simulink model "OL_HiLData"  (R2015b)
settings: Solver=FixedStepDiscrete  StartTime=0.0  StopTime=stop_time  FixedStep=step_size  RelTol=1e-3
values from neighbouring files (symbols this model uses):
  step_size = 0.1    [loadCalib.m]
  stop_time = 660    [run_test_cases.m]
undefined symbols (not defined in the file or in its folder): canChannel
libraries: canmsglib x62, canlib x29, realtime_pacer_lib x1
(part 3 of 4)

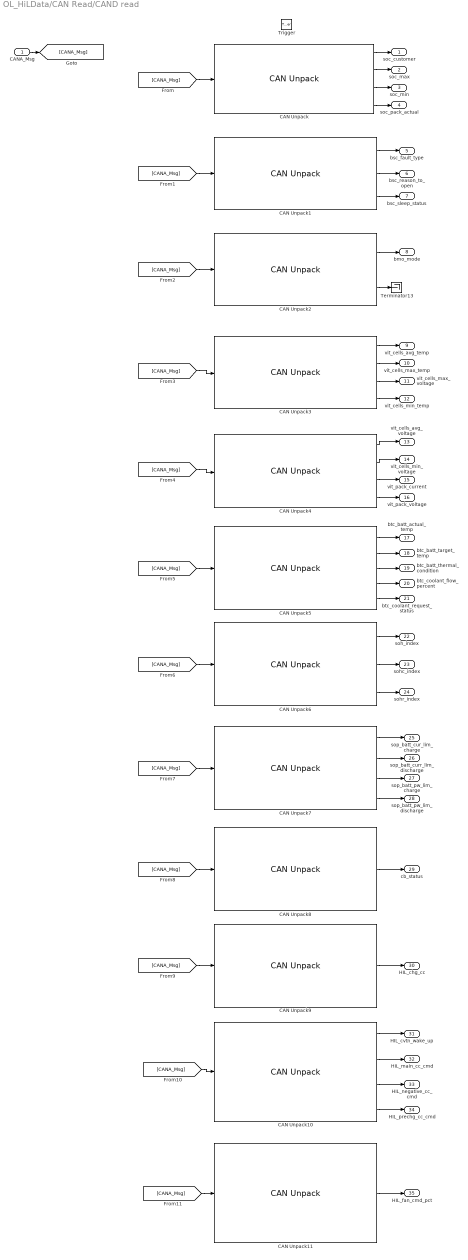
== system OL_HiLData/CAN Read/CAND read ==
  CANA_Msg : Inport
  Trigger : TriggerPort  TriggerType=function-call  PortDimensions=1
  CAN Unpack : canmsglib/CAN Unpack  CANdbFile=D:\Projects\BMS\P006n\08_Work_in_progress\Repo_Sync_folder\OpenLoopDataSendCAN\VEHdb.dbc  MsgList=soc_info  MsgName=soc_info  MsgIDType=Standard (11-bit identifier)  MsgIdentifier=40  MsgLength=8  SignalInfo=soc_customer$8$16$2$2$1$0$1.000000e-02$0$0$100$#soc_max$56$16$2$2$1$0$1.000000e-02$0$0$100$#soc_min$40$16$2$2$1$0$1.000000e-02$0$0$100$#soc_pack_actual$24$16$2$2$1$0$1.000000e-02$0$0$100$#  NSignals=4  IDPort=off  TimestampPort=off  ErrorPort=off  RemotePort=off  LengthPort=off  StatusPort=off  StartBits=str2num('[int32(8);int32(56);int32(40);int32(24)]')  SignalSizes=str2num('[int32(16);int32(16);int32(16);int32(16)]')  ByteOrders=str2num('[int32(2);int32(2);int32(2);int32(2)]')  DataTypes=str2num('[int32(2);int32(2);int32(2);int32(2)]')  MultiplexTypes=str2num('[int32(1);int32(1);int32(1);int32(1)]')  MultiplexValues=str2num('[double(0);double(0);double(0);double(0)]')  Factors=str2num('[double(1.000000e-02);double(1.000000e-02);double(1.000000e-02);double(1.000000e-02)]')  Offsets=str2num('[double(0);double(0);double(0);double(0)]')  Minimums=str2num('[double(0);double(0);double(0);double(0)]')  Maximums=str2num('[double(100);double(100);double(100);double(100)]')
      settings: DataFormat=CANdb specified signals
  CAN Unpack1 : canmsglib/CAN Unpack  CANdbFile=D:\Projects\BMS\P006n\08_Work_in_progress\Repo_Sync_folder\OpenLoopDataSendCAN\VEHdb.dbc  MsgList=bsc_info  MsgName=bsc_info  MsgIDType=Standard (11-bit identifier)  MsgIdentifier=41  MsgLength=8  SignalInfo=bsc_fault_type$8$8$2$2$1$0$1$0$0$20$#bsc_reason_to_open$0$8$2$2$1$0$1$0$0$20$#bsc_sleep_status$23$1$2$2$1$0$1$0$0$1$#  NSignals=3  IDPort=off  TimestampPort=off  ErrorPort=off  RemotePort=off  LengthPort=off  StatusPort=off  StartBits=str2num('[int32(8);int32(0);int32(23)]')  SignalSizes=str2num('[int32(8);int32(8);int32(1)]')  ByteOrders=str2num('[int32(2);int32(2);int32(2)]')  DataTypes=str2num('[int32(2);int32(2);int32(2)]')  MultiplexTypes=str2num('[int32(1);int32(1);int32(1)]')  MultiplexValues=str2num('[double(0);double(0);double(0)]')  Factors=str2num('[double(1);double(1);double(1)]')  Offsets=str2num('[double(0);double(0);double(0)]')  Minimums=str2num('[double(0);double(0);double(0)]')  Maximums=str2num('[double(20);double(20);double(1)]')
      settings: DataFormat=CANdb specified signals
  CAN Unpack10 : canmsglib/CAN Unpack  CANdbFile=D:\Projects\BMS\P006n\08_Work_in_progress\Repo_Sync_folder\OpenLoopDataSendCAN\BMSdb.dbc  MsgList=contactor_cmds  MsgName=contactor_cmds  MsgIDType=Standard (11-bit identifier)  MsgIdentifier=38  MsgLength=8  SignalInfo=cvtn_wake_up$4$1$2$2$1$0$1$0$0$1$#main_contactor_cmd$7$1$2$2$1$0$1$0$0$1$#negative_contactor_cmd$5$1$2$2$1$0$1$0$0$1$#precharge_contactor_cmd$6$1$2$2$1$0$1$0$0$1$#  NSignals=4  IDPort=off  TimestampPort=off  ErrorPort=off  RemotePort=off  LengthPort=off  StatusPort=off  StartBits=str2num('[int32(4);int32(7);int32(5);int32(6)]')  SignalSizes=str2num('[int32(1);int32(1);int32(1);int32(1)]')  ByteOrders=str2num('[int32(2);int32(2);int32(2);int32(2)]')  DataTypes=str2num('[int32(2);int32(2);int32(2);int32(2)]')  MultiplexTypes=str2num('[int32(1);int32(1);int32(1);int32(1)]')  MultiplexValues=str2num('[double(0);double(0);double(0);double(0)]')  Factors=str2num('[double(1);double(1);double(1);double(1)]')  Offsets=str2num('[double(0);double(0);double(0);double(0)]')  Minimums=str2num('[double(0);double(0);double(0);double(0)]')  Maximums=str2num('[double(1);double(1);double(1);double(1)]')
      settings: DataFormat=CANdb specified signals
  CAN Unpack11 : canmsglib/CAN Unpack  CANdbFile=D:\Projects\BMS\P006n\08_Work_in_progress\Repo_Sync_folder\OpenLoopDataSendCAN\BMSdb.dbc  MsgList=fan_cmd  MsgName=fan_cmd  MsgIDType=Standard (11-bit identifier)  MsgIdentifier=39  MsgLength=8  SignalInfo=fan_cmd_pct$14$10$2$2$1$0$1.000000e-01$0$0$100$#  NSignals=1  IDPort=off  TimestampPort=off  ErrorPort=off  RemotePort=off  LengthPort=off  StatusPort=off  StartBits=str2num('[int32(14)]')  SignalSizes=str2num('[int32(10)]')  ByteOrders=str2num('[int32(2)]')  DataTypes=str2num('[int32(2)]')  MultiplexTypes=str2num('[int32(1)]')  MultiplexValues=str2num('[double(0)]')  Factors=str2num('[double(1.000000e-01)]')  Offsets=str2num('[double(0)]')  Minimums=str2num('[double(0)]')  Maximums=str2num('[double(100)]')
      settings: DataFormat=CANdb specified signals
  CAN Unpack2 : canmsglib/CAN Unpack  CANdbFile=D:\Projects\BMS\P006n\08_Work_in_progress\Repo_Sync_folder\OpenLoopDataSendCAN\VEHdb.dbc  MsgList=bmo_info  MsgName=bmo_info  MsgIDType=Standard (11-bit identifier)  MsgIdentifier=48  MsgLength=8  SignalInfo=bmo_mode$0$8$2$2$1$0$1$0$0$10$#soc_rate_high$15$1$2$2$1$0$1$0$0$1$#  NSignals=2  IDPort=off  TimestampPort=off  ErrorPort=off  RemotePort=off  LengthPort=off  StatusPort=off  StartBits=str2num('[int32(0);int32(15)]')  SignalSizes=str2num('[int32(8);int32(1)]')  ByteOrders=str2num('[int32(2);int32(2)]')  DataTypes=str2num('[int32(2);int32(2)]')  MultiplexTypes=str2num('[int32(1);int32(1)]')  MultiplexValues=str2num('[double(0);double(0)]')  Factors=str2num('[double(1);double(1)]')  Offsets=str2num('[double(0);double(0)]')  Minimums=str2num('[double(0);double(0)]')  Maximums=str2num('[double(10);double(1)]')
      settings: DataFormat=CANdb specified signals
  CAN Unpack3 : canmsglib/CAN Unpack  CANdbFile=D:\Projects\BMS\P006n\08_Work_in_progress\Repo_Sync_folder\OpenLoopDataSendCAN\VEHdb.dbc  MsgList=vit_info1  MsgName=vit_info1  MsgIDType=Standard (11-bit identifier)  MsgIdentifier=49  MsgLength=8  SignalInfo=vit_cells_avg_temp$40$16$2$1$1$0$1.000000e-02$0$-100$120$#vit_cells_max_temp$8$16$2$1$1$0$1.000000e-02$0$-100$120$#vit_cells_max_voltage$56$16$2$2$1$0$1.000000e-02$0$0$5$#vit_cells_min_temp$24$16$2$1$1$0$1.000000e-02$0$-100$120$#  NSignals=4  IDPort=off  TimestampPort=off  ErrorPort=off  RemotePort=off  LengthPort=off  StatusPort=off  StartBits=str2num('[int32(40);int32(8);int32(56);int32(24)]')  SignalSizes=str2num('[int32(16);int32(16);int32(16);int32(16)]')  ByteOrders=str2num('[int32(2);int32(2);int32(2);int32(2)]')  DataTypes=str2num('[int32(1);int32(1);int32(2);int32(1)]')  MultiplexTypes=str2num('[int32(1);int32(1);int32(1);int32(1)]')  MultiplexValues=str2num('[double(0);double(0);double(0);double(0)]')  Factors=str2num('[double(1.000000e-02);double(1.000000e-02);double(1.000000e-02);double(1.000000e-02)]')  Offsets=str2num('[double(0);double(0);double(0);double(0)]')  Minimums=str2num('[double(-100);double(-100);double(0);double(-100)]')  Maximums=str2num('[double(120);double(120);double(5);double(120)]')
      settings: DataFormat=CANdb specified signals
  CAN Unpack4 : canmsglib/CAN Unpack  CANdbFile=D:\Projects\BMS\P006n\08_Work_in_progress\Repo_Sync_folder\OpenLoopDataSendCAN\VEHdb.dbc  MsgList=vit_info2  MsgName=vit_info2  MsgIDType=Standard (11-bit identifier)  MsgIdentifier=50  MsgLength=8  SignalInfo=vit_cells_avg_voltage$24$16$2$2$1$0$1.000000e-02$0$0$5$#vit_cells_min_voltage$8$16$2$2$1$0$1.000000e-02$0$0$5$#vit_pack_current$56$16$2$1$1$0$1.000000e-02$0$-300$300$#vit_pack_voltage$40$16$2$2$1$0$1.000000e-02$0$0$200$#  NSignals=4  IDPort=off  TimestampPort=off  ErrorPort=off  RemotePort=off  LengthPort=off  StatusPort=off  StartBits=str2num('[int32(24);int32(8);int32(56);int32(40)]')  SignalSizes=str2num('[int32(16);int32(16);int32(16);int32(16)]')  ByteOrders=str2num('[int32(2);int32(2);int32(2);int32(2)]')  DataTypes=str2num('[int32(2);int32(2);int32(1);int32(2)]')  MultiplexTypes=str2num('[int32(1);int32(1);int32(1);int32(1)]')  MultiplexValues=str2num('[double(0);double(0);double(0);double(0)]')  Factors=str2num('[double(1.000000e-02);double(1.000000e-02);double(1.000000e-02);double(1.000000e-02)]')  Offsets=str2num('[double(0);double(0);double(0);double(0)]')  Minimums=str2num('[double(0);double(0);double(-300);double(0)]')  Maximums=str2num('[double(5);double(5);double(300);double(200)]')
      settings: DataFormat=CANdb specified signals
  CAN Unpack5 : canmsglib/CAN Unpack  CANdbFile=D:\Projects\BMS\P006n\08_Work_in_progress\Repo_Sync_folder\OpenLoopDataSendCAN\VEHdb.dbc  MsgList=btc_info  MsgName=btc_info  MsgIDType=Standard (11-bit identifier)  MsgIdentifier=51  MsgLength=8  SignalInfo=btc_batt_actual_temp$16$16$2$1$1$0$5.000000e-01$0$-50$80$#btc_batt_target_temp$40$16$2$1$1$0$5.000000e-01$0$-50$80$#btc_batt_thermal_condition$6$1$2$2$1$0$1$0$0$1$#btc_coolant_flow_percent$24$8$2$2$1$0$1$0$0$100$#btc_coolant_request_status$7$1$2$2$1$0$1$0$0$1$#  NSignals=5  IDPort=off  TimestampPort=off  ErrorPort=off  RemotePort=off  LengthPort=off  StatusPort=off  StartBits=str2num('[int32(16);int32(40);int32(6);int32(24);int32(7)]')  SignalSizes=str2num('[int32(16);int32(16);int32(1);int32(8);int32(1)]')  ByteOrders=str2num('[int32(2);int32(2);int32(2);int32(2);int32(2)]')  DataTypes=str2num('[int32(1);int32(1);int32(2);int32(2);int32(2)]')  MultiplexTypes=str2num('[int32(1);int32(1);int32(1);int32(1);int32(1)]')  MultiplexValues=str2num('[double(0);double(0);double(0);double(0);double(0)]')  Factors=str2num('[double(5.000000e-01);double(5.000000e-01);double(1);double(1);double(1)]')  Offsets=str2num('[double(0);double(0);double(0);double(0);double(0)]')  Minimums=str2num('[double(-50);double(-50);double(0);double(0);double(0)]')  Maximums=str2num('[double(80);double(80);double(1);double(100);double(1)]')
      settings: DataFormat=CANdb specified signals
  CAN Unpack6 : canmsglib/CAN Unpack  CANdbFile=D:\Projects\BMS\P006n\08_Work_in_progress\Repo_Sync_folder\OpenLoopDataSendCAN\VEHdb.dbc  MsgList=soh_info  MsgName=soh_info  MsgIDType=Standard (11-bit identifier)  MsgIdentifier=52  MsgLength=8  SignalInfo=soh_index$8$16$2$2$1$0$1.000000e-02$0$0$100$#sohc_index$40$16$2$2$1$0$1.000000e-02$0$0$100$#sohr_index$24$16$2$2$1$0$1.000000e-02$0$0$100$#  NSignals=3  IDPort=off  TimestampPort=off  ErrorPort=off  RemotePort=off  LengthPort=off  StatusPort=off  StartBits=str2num('[int32(8);int32(40);int32(24)]')  SignalSizes=str2num('[int32(16);int32(16);int32(16)]')  ByteOrders=str2num('[int32(2);int32(2);int32(2)]')  DataTypes=str2num('[int32(2);int32(2);int32(2)]')  MultiplexTypes=str2num('[int32(1);int32(1);int32(1)]')  MultiplexValues=str2num('[double(0);double(0);double(0)]')  Factors=str2num('[double(1.000000e-02);double(1.000000e-02);double(1.000000e-02)]')  Offsets=str2num('[double(0);double(0);double(0)]')  Minimums=str2num('[double(0);double(0);double(0)]')  Maximums=str2num('[double(100);double(100);double(100)]')
      settings: DataFormat=CANdb specified signals
  CAN Unpack7 : canmsglib/CAN Unpack  CANdbFile=D:\Projects\BMS\P006n\08_Work_in_progress\Repo_Sync_folder\OpenLoopDataSendCAN\VEHdb.dbc  MsgList=sop_info  MsgName=sop_info  MsgIDType=Standard (11-bit identifier)  MsgIdentifier=53  MsgLength=8  SignalInfo=sop_batt_curr_lim_charge$40$16$2$2$1$0$5.000000e-02$0$0$512$#sop_batt_curr_lim_discharge$56$16$2$2$1$0$5.000000e-02$0$0$512$#sop_batt_pw_lim_charge$8$16$2$2$1$0$4$0$0$256000$#sop_batt_pw_lim_discharge$24$16$2$2$1$0$4$0$0$256000$#  NSignals=4  IDPort=off  TimestampPort=off  ErrorPort=off  RemotePort=off  LengthPort=off  StatusPort=off  StartBits=str2num('[int32(40);int32(56);int32(8);int32(24)]')  SignalSizes=str2num('[int32(16);int32(16);int32(16);int32(16)]')  ByteOrders=str2num('[int32(2);int32(2);int32(2);int32(2)]')  DataTypes=str2num('[int32(2);int32(2);int32(2);int32(2)]')  MultiplexTypes=str2num('[int32(1);int32(1);int32(1);int32(1)]')  MultiplexValues=str2num('[double(0);double(0);double(0);double(0)]')  Factors=str2num('[double(5.000000e-02);double(5.000000e-02);double(4);double(4)]')  Offsets=str2num('[double(0);double(0);double(0);double(0)]')  Minimums=str2num('[double(0);double(0);double(0);double(0)]')  Maximums=str2num('[double(512);double(512);double(256000);double(256000)]')
      settings: DataFormat=CANdb specified signals
  CAN Unpack8 : canmsglib/CAN Unpack  CANdbFile=D:\Projects\BMS\P006n\08_Work_in_progress\Repo_Sync_folder\OpenLoopDataSendCAN\VEHdb.dbc  MsgList=cb_info  MsgName=cb_info  MsgIDType=Standard (11-bit identifier)  MsgIdentifier=54  MsgLength=8  SignalInfo=cb_status$7$1$2$2$1$0$1$0$0$1$#  NSignals=1  IDPort=off  TimestampPort=off  ErrorPort=off  RemotePort=off  LengthPort=off  StatusPort=off  StartBits=str2num('[int32(7)]')  SignalSizes=str2num('[int32(1)]')  ByteOrders=str2num('[int32(2)]')  DataTypes=str2num('[int32(2)]')  MultiplexTypes=str2num('[int32(1)]')  MultiplexValues=str2num('[double(0)]')  Factors=str2num('[double(1)]')  Offsets=str2num('[double(0)]')  Minimums=str2num('[double(0)]')  Maximums=str2num('[double(1)]')
      settings: DataFormat=CANdb specified signals
  CAN Unpack9 : canmsglib/CAN Unpack  CANdbFile=D:\Projects\BMS\P006n\08_Work_in_progress\Repo_Sync_folder\OpenLoopDataSendCAN\VEHdb.dbc  MsgList=socket_charging_contactor  MsgName=socket_charging_contactor  MsgIDType=Standard (11-bit identifier)  MsgIdentifier=55  MsgLength=8  SignalInfo=charger_contactor$7$1$2$2$1$0$1$0$0$1$#  NSignals=1  IDPort=off  TimestampPort=off  ErrorPort=off  RemotePort=off  LengthPort=off  StatusPort=off  StartBits=str2num('[int32(7)]')  SignalSizes=str2num('[int32(1)]')  ByteOrders=str2num('[int32(2)]')  DataTypes=str2num('[int32(2)]')  MultiplexTypes=str2num('[int32(1)]')  MultiplexValues=str2num('[double(0)]')  Factors=str2num('[double(1)]')  Offsets=str2num('[double(0)]')  Minimums=str2num('[double(0)]')  Maximums=str2num('[double(1)]')
      settings: DataFormat=CANdb specified signals
  Terminator13 : Terminator
  soc_customer : Outport
  soc_max : Outport  Port=2
  soc_min : Outport  Port=3
  soc_pack_actual : Outport  Port=4
  bsc_fault_type : Outport  Port=5
  bsc_reason_to_open : Outport  Port=6
  bsc_sleep_status : Outport  Port=7
  bmo_mode : Outport  Port=8
  vit_cells_avg_temp : Outport  Port=9
  vit_cells_max_temp : Outport  Port=10
  vit_cells_max_voltage : Outport  Port=11
  vit_cells_min_temp : Outport  Port=12
  vit_cells_avg_voltage : Outport  Port=13
  vit_cells_min_voltage : Outport  Port=14
  vit_pack_current : Outport  Port=15
  vit_pack_voltage : Outport  Port=16
  btc_batt_actual_temp : Outport  Port=17
  btc_batt_target_temp : Outport  Port=18
  btc_batt_thermal_condition : Outport  Port=19
  btc_coolant_flow_percent : Outport  Port=20
  btc_coolant_request_status : Outport  Port=21
  soh_index : Outport  Port=22
  sohc_index : Outport  Port=23
  sohr_index : Outport  Port=24
  sop_batt_cur_lim_charge : Outport  Port=25
  sop_batt_curr_lim_discharge : Outport  Port=26
  sop_batt_pw_lim_charge : Outport  Port=27
  sop_batt_pw_lim_discharge : Outport  Port=28
  cb_status : Outport  Port=29
  HIL_chg_cc : Outport  Port=30
  HIL_cvtn_wake_up : Outport  Port=31
  HIL_main_cc_cmd : Outport  Port=32
  HIL_negative_cc_cmd : Outport  Port=33
  HIL_prechg_cc_cmd : Outport  Port=34
  HIL_fan_cmd_pct : Outport  Port=35
  wires:
  CAN Unpack/1 -> soc_customer/1
  CAN Unpack/2 -> soc_max/1
  CAN Unpack/3 -> soc_min/1
  CAN Unpack/4 -> soc_pack_actual/1
  CANA_Msg/1 -> [CANA_Msg]
  [CANA_Msg] -> CAN Unpack/1
  [CANA_Msg] -> CAN Unpack1/1
  CAN Unpack1/1 -> bsc_fault_type/1
  CAN Unpack1/2 -> bsc_reason_to_open/1
  CAN Unpack1/3 -> bsc_sleep_status/1
  [CANA_Msg] -> CAN Unpack2/1
  CAN Unpack2/1 -> bmo_mode/1
  [CANA_Msg] -> CAN Unpack3/1
  CAN Unpack3/1 -> vit_cells_avg_temp/1
  CAN Unpack3/2 -> vit_cells_max_temp/1
  CAN Unpack3/3 -> vit_cells_max_voltage/1
  CAN Unpack3/4 -> vit_cells_min_temp/1
  [CANA_Msg] -> CAN Unpack4/1
  CAN Unpack4/1 -> vit_cells_avg_voltage/1
  CAN Unpack4/2 -> vit_cells_min_voltage/1
  CAN Unpack4/3 -> vit_pack_current/1
  CAN Unpack4/4 -> vit_pack_voltage/1
  [CANA_Msg] -> CAN Unpack5/1
  CAN Unpack5/1 -> btc_batt_actual_temp/1
  CAN Unpack5/2 -> btc_batt_target_temp/1
  CAN Unpack5/3 -> btc_batt_thermal_condition/1
  CAN Unpack5/4 -> btc_coolant_flow_percent/1
  CAN Unpack5/5 -> btc_coolant_request_status/1
  [CANA_Msg] -> CAN Unpack6/1
  CAN Unpack6/1 -> soh_index/1
  [CANA_Msg] -> CAN Unpack7/1
  CAN Unpack7/1 -> sop_batt_cur_lim_charge/1
  CAN Unpack7/2 -> sop_batt_curr_lim_discharge/1
  CAN Unpack7/3 -> sop_batt_pw_lim_charge/1
  CAN Unpack7/4 -> sop_batt_pw_lim_discharge/1
  [CANA_Msg] -> CAN Unpack8/1
  CAN Unpack8/1 -> cb_status/1
  CAN Unpack6/3 -> sohr_index/1
  CAN Unpack6/2 -> sohc_index/1
  [CANA_Msg] -> CAN Unpack9/1
  CAN Unpack9/1 -> HIL_chg_cc/1
  [CANA_Msg] -> CAN Unpack10/1
  CAN Unpack10/1 -> HIL_cvtn_wake_up/1
  CAN Unpack10/2 -> HIL_main_cc_cmd/1
  CAN Unpack10/3 -> HIL_negative_cc_cmd/1
  CAN Unpack10/4 -> HIL_prechg_cc_cmd/1
  [CANA_Msg] -> CAN Unpack11/1
  CAN Unpack11/1 -> HIL_fan_cmd_pct/1
  CAN Unpack2/2 -> Terminator13/1

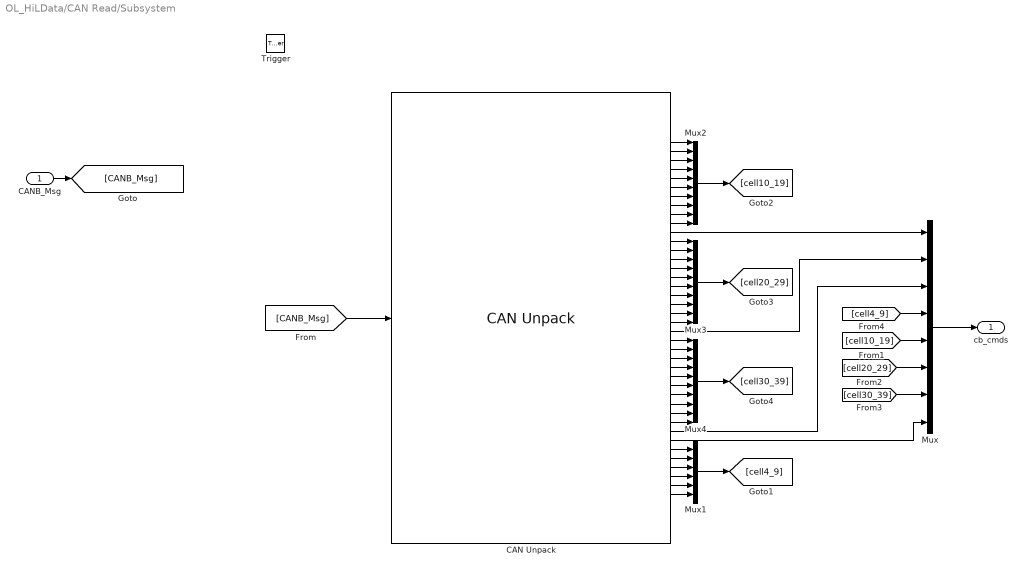
== system OL_HiLData/CAN Read/Subsystem ==
  CANB_Msg : Inport
  Trigger : TriggerPort  TriggerType=function-call  PortDimensions=1
  CAN Unpack : canmsglib/CAN Unpack  CANdbFile=D:\Projects\BMS\P006n\08_Work_in_progress\Repo_Sync_folder\OpenLoopDataSendCAN\BMSdb.dbc  MsgList=cell_bal_cmd  MsgName=cell_bal_cmd  MsgIDType=Standard (11-bit identifier)  MsgIdentifier=34  MsgLength=8  SignalInfo=cell10_cb_cmd$14$1$2$2$1$0$1$0$0$1$#cell11_cb_cmd$13$1$2$2$1$0$1$0$0$1$#cell12_cb_cmd$12$1$2$2$1$0$1$0$0$1$#cell13_cb_cmd$11$1$2$2$1$0$1$0$0$1$#cell14_cb_cmd$10$1$2$2$1$0$1$0$0$1$#cell15_cb_cmd$9$1$2$2$1$0$1$0$0$1$#cell16_cb_cmd$8$1$2$2$1$0$1$0$0$1$#cell17_cb_cmd$23$1$2$2$1$0$1$0$0$1$#cell18_cb_cmd$22$1$2$2$1$0$1$0$0$1$#cell19_cb_cmd$21$1$2$2$1$0$1$0$0$1$#cell1_cb_cmd$7$1$2$2$1$0$1$0$0$1$#cell20_cb_cmd$20$1$2$2$1$0$1$0$0$1$#cell21_cb_cmd$19$1$2$2$1$0$1$0$0$1$#cell22_cb_cmd$18$1$2$2$1$0$1$0$0$1$#cell23_cb_cmd$17$1$2$2$1$0$1$0$0$1$#cell24_cb_cmd$16$1$2$2$1$0$1$0$0$1$#cell25_cb_cmd$31$1$2$2$1$0$1$0$0$1$#cell26_cb_cmd$30$1$2$2$1$0$1$0$0$1$#cell27_cb_cmd$29$1$2$2$1$0$1$0$0$1$#cell28_cb_cmd$28$1$2$2$1$0$1$0$0$1$#cell29_cb_cmd$27$1$2$2$1$0$1$0$0$1$#cell2_cb_cmd$6$1$2$2$1$0$1$0$0$1$#cell30_cb_cmd$26$1$2$2$1$0$1$0$0$1$#cell31_cb_cmd$25$1$2$2$1$0$1$0$0$1$#cell32_cb_cmd$24$1$2$2$1$0$1$0$0$1$#cell33_cb_cmd$39$1$2$2$1$0$1$0$0$1$#cell34_cb_cmd$38$1$2$2$1$0$1$0$0$1$#cell35_cb_cmd$37$1$2$2$1$0$1$0$0$1$#cell36_cb_cmd$36$1$2$2$1$0$1$0$0$1$#cell37_cb_cmd$35$1$2$2$1$0$1$0$0$1$#cell38_cb_cmd$34$1$2$2$1$0$1$0$0$1$#cell39_cb_cmd$33$1$2$2$1$0$1$0$0$1$#cell3_cb_cmd$5$1$2$2$1$0$1$0$0$1$#cell40_cb_cmd$32$1$2$2$1$0$1$0$0$1$#cell4_cb_cmd$4$1$2$2$1$0$1$0$0$1$#cell5_cb_cmd$3$1$2$2$1$0$1$0$0$1$#cell6_cb_cmd$2$1$2$2$1$0$1$0$0$1$#cell7_cb_cmd$1$1$2$2$1$0$1$0$0$1$#cell8_cb_cmd$0$1$2$2$1$0$1$0$0$1$#cell9_cb_cmd$15$1$2$2$1$0$1$0$0$1$#  NSignals=40  IDPort=off  TimestampPort=off  ErrorPort=off  RemotePort=off  LengthPort=off  StatusPort=off  StartBits=str2num('[int32(14);int32(13);int32(12);int32(11);int32(10);int32(9);int32(8);int32(23);int32(22);int32(21);int32(7);int32(20);int32(19);int32(18);int32(17);int32(16);int32(31);int32(30);int32(29);int32(28);int32(27);int32(6);int32(26);int32(25);int32(24);int32(39);int32(38);int32(37);int32(36);int32(35);int32(34);int32(33);int32(5);int32(32);int32(4);int32(3);int32(2);int32(1);int32(0);int32(15)]')  SignalSizes=str2num('[int32(1);int32(1);int32(1);int32(1);int32(1);int32(1);int32(1);int32(1);int32(1);int32(1);int32(1);int32(1);int32(1);int32(1);int32(1);int32(1);int32(1);int32(1);int32(1);int32(1);int32(1);int32(1);int32(1);int32(1);int32(1);int32(1);int32(1);int32(1);int32(1);int32(1);int32(1);int32(1);int32(1);int32(1);int32(1);int32(1);int32(1);int32(1);int32(1);int32(1)]')  ByteOrders=str2num('[int32(2);int32(2);int32(2);int32(2);int32(2);int32(2);int32(2);int32(2);int32(2);int32(2);int32(2);int32(2);int32(2);int32(2);int32(2);int32(2);int32(2);int32(2);int32(2);int32(2);int32(2);int32(2);int32(2);int32(2);int32(2);int32(2);int32(2);int32(2);int32(2);int32(2);int32(2);int32(2);int32(2);int32(2);int32(2);int32(2);int32(2);int32(2);int32(2);int32(2)]')  DataTypes=str2num('[int32(2);int32(2);int32(2);int32(2);int32(2);int32(2);int32(2);int32(2);int32(2);int32(2);int32(2);int32(2);int32(2);int32(2);int32(2);int32(2);int32(2);int32(2);int32(2);int32(2);int32(2);int32(2);int32(2);int32(2);int32(2);int32(2);int32(2);int32(2);int32(2);int32(2);int32(2);int32(2);int32(2);int32(2);int32(2);int32(2);int32(2);int32(2);int32(2);int32(2)]')  MultiplexTypes=str2num('[int32(1);int32(1);int32(1);int32(1);int32(1);int32(1);int32(1);int32(1);int32(1);int32(1);int32(1);int32(1);int32(1);int32(1);int32(1);int32(1);int32(1);int32(1);int32(1);int32(1);int32(1);int32(1);int32(1);int32(1);int32(1);int32(1);int32(1);int32(1);int32(1);int32(1);int32(1);int32(1);int32(1);int32(1);int32(1);int32(1);int32(1);int32(1);int32(1);int32(1)]')  MultiplexValues=str2num('[double(0);double(0);double(0);double(0);double(0);double(0);double(0);double(0);double(0);double(0);double(0);double(0);double(0);double(0);double(0);double(0);double(0);double(0);double(0);double(0);double(0);double(0);double(0);double(0);double(0);double(0);double(0);double(0);double(0);double(0);double(0);double(0);double(0);double(0);double(0);double(0);double(0);double(0);double(0);double(0)]')  Factors=str2num('[double(1);double(1);double(1);double(1);double(1);double(1);double(1);double(1);double(1);double(1);double(1);double(1);double(1);double(1);double(1);double(1);double(1);double(1);double(1);double(1);double(1);double(1);double(1);double(1);double(1);double(1);double(1);double(1);double(1);double(1);double(1);double(1);double(1);double(1);double(1);double(1);double(1);double(1);double(1);double(1)]')  Offsets=str2num('[double(0);double(0);double(0);double(0);double(0);double(0);double(0);double(0);double(0);double(0);double(0);double(0);double(0);double(0);double(0);double(0);double(0);double(0);double(0);double(0);double(0);double(0);double(0);double(0);double(0);double(0);double(0);double(0);double(0);double(0);double(0);double(0);double(0);double(0);double(0);double(0);double(0);double(0);double(0);double(0)]')  Minimums=str2num('[double(0);double(0);double(0);double(0);double(0);double(0);double(0);double(0);double(0);double(0);double(0);double(0);double(0);double(0);double(0);double(0);double(0);double(0);double(0);double(0);double(0);double(0);double(0);double(0);double(0);double(0);double(0);double(0);double(0);double(0);double(0);double(0);double(0);double(0);double(0);double(0);double(0);double(0);double(0);double(0)]')  Maximums=str2num('[double(1);double(1);double(1);double(1);double(1);double(1);double(1);double(1);double(1);double(1);double(1);double(1);double(1);double(1);double(1);double(1);double(1);double(1);double(1);double(1);double(1);double(1);double(1);double(1);double(1);double(1);double(1);double(1);double(1);double(1);double(1);double(1);double(1);double(1);double(1);double(1);double(1);double(1);double(1);double(1)]')
      settings: DataFormat=CANdb specified signals
  Mux : Mux  Inputs=8
  Mux1 : Mux  Inputs=6
  Mux2 : Mux  Inputs=10
  Mux3 : Mux  Inputs=10
  Mux4 : Mux  Inputs=10
  cb_cmds : Outport
  wires:
  CANB_Msg/1 -> [CANB_Msg]
  [CANB_Msg] -> CAN Unpack/1
  CAN Unpack/35 -> Mux1/1
  CAN Unpack/36 -> Mux1/2
  CAN Unpack/37 -> Mux1/3
  CAN Unpack/38 -> Mux1/4
  CAN Unpack/39 -> Mux1/5
  CAN Unpack/40 -> Mux1/6
  CAN Unpack/1 -> Mux2/1
  CAN Unpack/2 -> Mux2/2
  CAN Unpack/3 -> Mux2/3
  CAN Unpack/4 -> Mux2/4
  CAN Unpack/5 -> Mux2/5
  CAN Unpack/6 -> Mux2/6
  CAN Unpack/7 -> Mux2/7
  CAN Unpack/8 -> Mux2/8
  CAN Unpack/9 -> Mux2/9
  CAN Unpack/10 -> Mux2/10
  Mux1/1 -> [cell4_9]
  Mux2/1 -> [cell10_19]
  CAN Unpack/12 -> Mux3/1
  CAN Unpack/13 -> Mux3/2
  CAN Unpack/14 -> Mux3/3
  CAN Unpack/15 -> Mux3/4
  CAN Unpack/16 -> Mux3/5
  CAN Unpack/17 -> Mux3/6
  CAN Unpack/18 -> Mux3/7
  CAN Unpack/19 -> Mux3/8
  CAN Unpack/20 -> Mux3/9
  CAN Unpack/21 -> Mux3/10
  Mux3/1 -> [cell20_29]
  CAN Unpack/23 -> Mux4/1
  CAN Unpack/24 -> Mux4/2
  CAN Unpack/25 -> Mux4/3
  CAN Unpack/26 -> Mux4/4
  CAN Unpack/27 -> Mux4/5
  CAN Unpack/28 -> Mux4/6
  CAN Unpack/29 -> Mux4/7
  CAN Unpack/30 -> Mux4/8
  CAN Unpack/31 -> Mux4/9
  CAN Unpack/32 -> Mux4/10
  Mux4/1 -> [cell30_39]
  CAN Unpack/11 -> Mux/1
  CAN Unpack/22 -> Mux/2
  CAN Unpack/33 -> Mux/3
  [cell4_9] -> Mux/4
  [cell10_19] -> Mux/5
  [cell20_29] -> Mux/6
  [cell30_39] -> Mux/7
  CAN Unpack/34 -> Mux/8
  Mux/1 -> cb_cmds/1

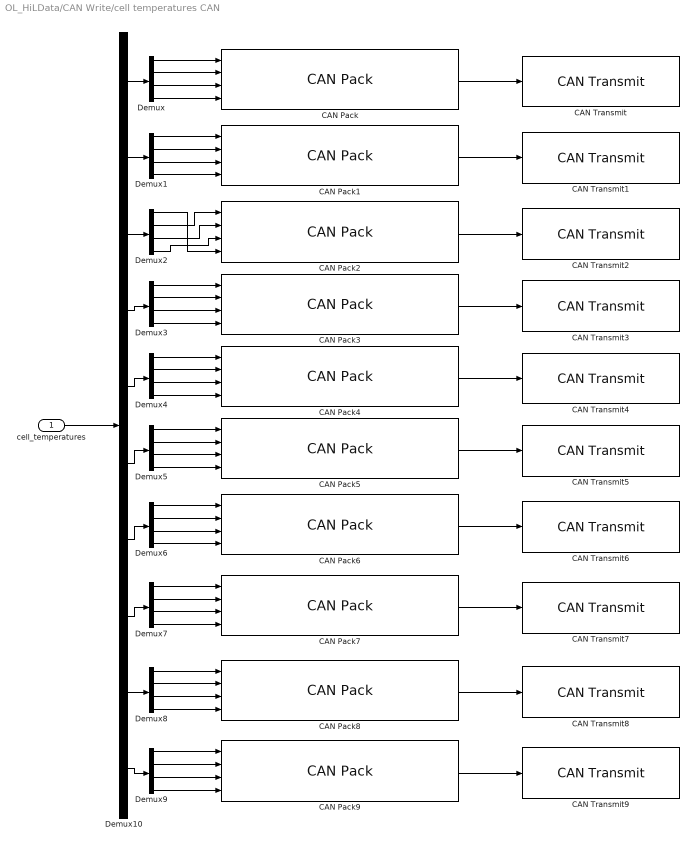
== system OL_HiLData/CAN Write/cell temperatures CAN ==
  cell_temperatures : Inport
  CAN Pack : canmsglib/CAN Pack  CANdbFile=D:\Projects\BMS\P006n\08_Work_in_progress\Repo_Sync_folder\OpenLoopDataSendCAN\BMSdb.dbc  MsgList=cell_temp_1_4  MsgName=cell_temp_1_4  MsgIDType=Standard (11-bit identifier)  MsgIdentifier=18  MsgLength=8  SignalInfo=cell1_temperature$8$16$2$2$1$0$1.000000e-03$-20$-20$80$#cell2_temperature$24$16$2$2$1$0$1.000000e-03$-20$-20$80$#cell3_temperature$40$16$2$2$1$0$1.000000e-03$-20$-20$80$#cell4_temperature$56$16$2$2$1$0$1.000000e-03$-20$-20$80$#  NSignals=4  StartBits=str2num('[int32(8);int32(24);int32(40);int32(56)]')  SignalSizes=str2num('[int32(16);int32(16);int32(16);int32(16)]')  ByteOrders=str2num('[int32(2);int32(2);int32(2);int32(2)]')  DataTypes=str2num('[int32(2);int32(2);int32(2);int32(2)]')  MultiplexTypes=str2num('[int32(1);int32(1);int32(1);int32(1)]')  MultiplexValues=str2num('[double(0);double(0);double(0);double(0)]')  Factors=str2num('[double(1.000000e-03);double(1.000000e-03);double(1.000000e-03);double(1.000000e-03)]')  Offsets=str2num('[double(-20);double(-20);double(-20);double(-20)]')  Minimums=str2num('[double(-20);double(-20);double(-20);double(-20)]')  Maximums=str2num('[double(80);double(80);double(80);double(80)]')  Remote=off
      settings: DataFormat=CANdb specified signals
  CAN Pack1 : canmsglib/CAN Pack  CANdbFile=D:\Projects\BMS\P006n\08_Work_in_progress\Repo_Sync_folder\OpenLoopDataSendCAN\BMSdb.dbc  MsgList=cell_temp_5_8  MsgName=cell_temp_5_8  MsgIDType=Standard (11-bit identifier)  MsgIdentifier=19  MsgLength=8  SignalInfo=cell5_temperature$8$16$2$2$1$0$1.000000e-03$-20$-20$80$#cell6_temperature$24$16$2$2$1$0$1.000000e-03$-20$-20$80$#cell7_temperature$40$16$2$2$1$0$1.000000e-03$-20$-20$80$#cell8_temperature$56$16$2$2$1$0$1.000000e-03$-20$-20$80$#  NSignals=4  StartBits=str2num('[int32(8);int32(24);int32(40);int32(56)]')  SignalSizes=str2num('[int32(16);int32(16);int32(16);int32(16)]')  ByteOrders=str2num('[int32(2);int32(2);int32(2);int32(2)]')  DataTypes=str2num('[int32(2);int32(2);int32(2);int32(2)]')  MultiplexTypes=str2num('[int32(1);int32(1);int32(1);int32(1)]')  MultiplexValues=str2num('[double(0);double(0);double(0);double(0)]')  Factors=str2num('[double(1.000000e-03);double(1.000000e-03);double(1.000000e-03);double(1.000000e-03)]')  Offsets=str2num('[double(-20);double(-20);double(-20);double(-20)]')  Minimums=str2num('[double(-20);double(-20);double(-20);double(-20)]')  Maximums=str2num('[double(80);double(80);double(80);double(80)]')  Remote=off
      settings: DataFormat=CANdb specified signals
  CAN Pack2 : canmsglib/CAN Pack  CANdbFile=D:\Projects\BMS\P006n\08_Work_in_progress\Repo_Sync_folder\OpenLoopDataSendCAN\BMSdb.dbc  MsgList=cell_temp_9_12  MsgName=cell_temp_9_12  MsgIDType=Standard (11-bit identifier)  MsgIdentifier=20  MsgLength=8  SignalInfo=cell10_temperature$24$16$2$2$1$0$1.000000e-03$-20$-20$80$#cell11_temperature$40$16$2$2$1$0$1.000000e-03$-20$-20$80$#cell12_temperature$56$16$2$2$1$0$1.000000e-03$-20$-20$80$#cell9_temperature$8$16$2$2$1$0$1.000000e-03$-20$-20$80$#  NSignals=4  StartBits=str2num('[int32(24);int32(40);int32(56);int32(8)]')  SignalSizes=str2num('[int32(16);int32(16);int32(16);int32(16)]')  ByteOrders=str2num('[int32(2);int32(2);int32(2);int32(2)]')  DataTypes=str2num('[int32(2);int32(2);int32(2);int32(2)]')  MultiplexTypes=str2num('[int32(1);int32(1);int32(1);int32(1)]')  MultiplexValues=str2num('[double(0);double(0);double(0);double(0)]')  Factors=str2num('[double(1.000000e-03);double(1.000000e-03);double(1.000000e-03);double(1.000000e-03)]')  Offsets=str2num('[double(-20);double(-20);double(-20);double(-20)]')  Minimums=str2num('[double(-20);double(-20);double(-20);double(-20)]')  Maximums=str2num('[double(80);double(80);double(80);double(80)]')  Remote=off
      settings: DataFormat=CANdb specified signals
  CAN Pack3 : canmsglib/CAN Pack  CANdbFile=D:\Projects\BMS\P006n\08_Work_in_progress\Repo_Sync_folder\OpenLoopDataSendCAN\BMSdb.dbc  MsgList=cell_temp_13_16  MsgName=cell_temp_13_16  MsgIDType=Standard (11-bit identifier)  MsgIdentifier=21  MsgLength=8  SignalInfo=cell13_temperature$8$16$2$2$1$0$1.000000e-03$-20$-20$80$#cell14_temperature$24$16$2$2$1$0$1.000000e-03$-20$-20$80$#cell15_temperature$40$16$2$2$1$0$1.000000e-03$-20$-20$80$#cell16_temperature$56$16$2$2$1$0$1.000000e-03$-20$-20$80$#  NSignals=4  StartBits=str2num('[int32(8);int32(24);int32(40);int32(56)]')  SignalSizes=str2num('[int32(16);int32(16);int32(16);int32(16)]')  ByteOrders=str2num('[int32(2);int32(2);int32(2);int32(2)]')  DataTypes=str2num('[int32(2);int32(2);int32(2);int32(2)]')  MultiplexTypes=str2num('[int32(1);int32(1);int32(1);int32(1)]')  MultiplexValues=str2num('[double(0);double(0);double(0);double(0)]')  Factors=str2num('[double(1.000000e-03);double(1.000000e-03);double(1.000000e-03);double(1.000000e-03)]')  Offsets=str2num('[double(-20);double(-20);double(-20);double(-20)]')  Minimums=str2num('[double(-20);double(-20);double(-20);double(-20)]')  Maximums=str2num('[double(80);double(80);double(80);double(80)]')  Remote=off
      settings: DataFormat=CANdb specified signals
  CAN Pack4 : canmsglib/CAN Pack  CANdbFile=D:\Projects\BMS\P006n\08_Work_in_progress\Repo_Sync_folder\OpenLoopDataSendCAN\BMSdb.dbc  MsgList=cell_temp_17_20  MsgName=cell_temp_17_20  MsgIDType=Standard (11-bit identifier)  MsgIdentifier=22  MsgLength=8  SignalInfo=cell17_temperature$8$16$2$2$1$0$1.000000e-03$-20$-20$80$#cell18_temperature$24$16$2$2$1$0$1.000000e-03$-20$-20$80$#cell19_temperature$40$16$2$2$1$0$1.000000e-03$-20$-20$80$#cell20_temperature$56$16$2$2$1$0$1.000000e-03$-20$-20$80$#  NSignals=4  StartBits=str2num('[int32(8);int32(24);int32(40);int32(56)]')  SignalSizes=str2num('[int32(16);int32(16);int32(16);int32(16)]')  ByteOrders=str2num('[int32(2);int32(2);int32(2);int32(2)]')  DataTypes=str2num('[int32(2);int32(2);int32(2);int32(2)]')  MultiplexTypes=str2num('[int32(1);int32(1);int32(1);int32(1)]')  MultiplexValues=str2num('[double(0);double(0);double(0);double(0)]')  Factors=str2num('[double(1.000000e-03);double(1.000000e-03);double(1.000000e-03);double(1.000000e-03)]')  Offsets=str2num('[double(-20);double(-20);double(-20);double(-20)]')  Minimums=str2num('[double(-20);double(-20);double(-20);double(-20)]')  Maximums=str2num('[double(80);double(80);double(80);double(80)]')  Remote=off
      settings: DataFormat=CANdb specified signals
  CAN Pack5 : canmsglib/CAN Pack  CANdbFile=D:\Projects\BMS\P006n\08_Work_in_progress\Repo_Sync_folder\OpenLoopDataSendCAN\BMSdb.dbc  MsgList=cell_temp_21_24  MsgName=cell_temp_21_24  MsgIDType=Standard (11-bit identifier)  MsgIdentifier=23  MsgLength=8  SignalInfo=cell21_temperature$8$16$2$2$1$0$1.000000e-03$-20$-20$80$#cell22_temperature$24$16$2$2$1$0$1.000000e-03$-20$-20$80$#cell23_temperature$40$16$2$2$1$0$1.000000e-03$-20$-20$80$#cell24_temperature$56$16$2$2$1$0$1.000000e-03$-20$-20$80$#  NSignals=4  StartBits=str2num('[int32(8);int32(24);int32(40);int32(56)]')  SignalSizes=str2num('[int32(16);int32(16);int32(16);int32(16)]')  ByteOrders=str2num('[int32(2);int32(2);int32(2);int32(2)]')  DataTypes=str2num('[int32(2);int32(2);int32(2);int32(2)]')  MultiplexTypes=str2num('[int32(1);int32(1);int32(1);int32(1)]')  MultiplexValues=str2num('[double(0);double(0);double(0);double(0)]')  Factors=str2num('[double(1.000000e-03);double(1.000000e-03);double(1.000000e-03);double(1.000000e-03)]')  Offsets=str2num('[double(-20);double(-20);double(-20);double(-20)]')  Minimums=str2num('[double(-20);double(-20);double(-20);double(-20)]')  Maximums=str2num('[double(80);double(80);double(80);double(80)]')  Remote=off
      settings: DataFormat=CANdb specified signals
  CAN Pack6 : canmsglib/CAN Pack  CANdbFile=D:\Projects\BMS\P006n\08_Work_in_progress\Repo_Sync_folder\OpenLoopDataSendCAN\BMSdb.dbc  MsgList=cell_temp_25_28  MsgName=cell_temp_25_28  MsgIDType=Standard (11-bit identifier)  MsgIdentifier=24  MsgLength=8  SignalInfo=cell25_temperature$8$16$2$2$1$0$1.000000e-03$-20$-20$80$#cell26_temperature$24$16$2$2$1$0$1.000000e-03$-20$-20$80$#cell27_temperature$40$16$2$2$1$0$1.000000e-03$-20$-20$80$#cell28_temperature$56$16$2$2$1$0$1.000000e-03$-20$-20$80$#  NSignals=4  StartBits=str2num('[int32(8);int32(24);int32(40);int32(56)]')  SignalSizes=str2num('[int32(16);int32(16);int32(16);int32(16)]')  ByteOrders=str2num('[int32(2);int32(2);int32(2);int32(2)]')  DataTypes=str2num('[int32(2);int32(2);int32(2);int32(2)]')  MultiplexTypes=str2num('[int32(1);int32(1);int32(1);int32(1)]')  MultiplexValues=str2num('[double(0);double(0);double(0);double(0)]')  Factors=str2num('[double(1.000000e-03);double(1.000000e-03);double(1.000000e-03);double(1.000000e-03)]')  Offsets=str2num('[double(-20);double(-20);double(-20);double(-20)]')  Minimums=str2num('[double(-20);double(-20);double(-20);double(-20)]')  Maximums=str2num('[double(80);double(80);double(80);double(80)]')  Remote=off
      settings: DataFormat=CANdb specified signals
  CAN Pack7 : canmsglib/CAN Pack  CANdbFile=D:\Projects\BMS\P006n\08_Work_in_progress\Repo_Sync_folder\OpenLoopDataSendCAN\BMSdb.dbc  MsgList=cell_temp_29_32  MsgName=cell_temp_29_32  MsgIDType=Standard (11-bit identifier)  MsgIdentifier=25  MsgLength=8  SignalInfo=cell29_temperature$8$16$2$2$1$0$1.000000e-03$-20$-20$80$#cell30_temperature$24$16$2$2$1$0$1.000000e-03$-20$-20$80$#cell31_temperature$40$16$2$2$1$0$1.000000e-03$-20$-20$80$#cell32_temperature$56$16$2$2$1$0$1.000000e-03$-20$-20$80$#  NSignals=4  StartBits=str2num('[int32(8);int32(24);int32(40);int32(56)]')  SignalSizes=str2num('[int32(16);int32(16);int32(16);int32(16)]')  ByteOrders=str2num('[int32(2);int32(2);int32(2);int32(2)]')  DataTypes=str2num('[int32(2);int32(2);int32(2);int32(2)]')  MultiplexTypes=str2num('[int32(1);int32(1);int32(1);int32(1)]')  MultiplexValues=str2num('[double(0);double(0);double(0);double(0)]')  Factors=str2num('[double(1.000000e-03);double(1.000000e-03);double(1.000000e-03);double(1.000000e-03)]')  Offsets=str2num('[double(-20);double(-20);double(-20);double(-20)]')  Minimums=str2num('[double(-20);double(-20);double(-20);double(-20)]')  Maximums=str2num('[double(80);double(80);double(80);double(80)]')  Remote=off
      settings: DataFormat=CANdb specified signals
  CAN Pack8 : canmsglib/CAN Pack  CANdbFile=D:\Projects\BMS\P006n\08_Work_in_progress\Repo_Sync_folder\OpenLoopDataSendCAN\BMSdb.dbc  MsgList=cell_temp_33_36  MsgName=cell_temp_33_36  MsgIDType=Standard (11-bit identifier)  MsgIdentifier=32  MsgLength=8  SignalInfo=cell33_temperature$8$16$2$2$1$0$1.000000e-03$-20$-20$80$#cell34_temperature$24$16$2$2$1$0$1.000000e-03$-20$-20$80$#cell35_temperature$40$16$2$2$1$0$1.000000e-03$-20$-20$80$#cell36_temperature$56$16$2$2$1$0$1.000000e-03$-20$-20$80$#  NSignals=4  StartBits=str2num('[int32(8);int32(24);int32(40);int32(56)]')  SignalSizes=str2num('[int32(16);int32(16);int32(16);int32(16)]')  ByteOrders=str2num('[int32(2);int32(2);int32(2);int32(2)]')  DataTypes=str2num('[int32(2);int32(2);int32(2);int32(2)]')  MultiplexTypes=str2num('[int32(1);int32(1);int32(1);int32(1)]')  MultiplexValues=str2num('[double(0);double(0);double(0);double(0)]')  Factors=str2num('[double(1.000000e-03);double(1.000000e-03);double(1.000000e-03);double(1.000000e-03)]')  Offsets=str2num('[double(-20);double(-20);double(-20);double(-20)]')  Minimums=str2num('[double(-20);double(-20);double(-20);double(-20)]')  Maximums=str2num('[double(80);double(80);double(80);double(80)]')  Remote=off
      settings: DataFormat=CANdb specified signals
  CAN Pack9 : canmsglib/CAN Pack  CANdbFile=D:\Projects\BMS\P006n\08_Work_in_progress\Repo_Sync_folder\OpenLoopDataSendCAN\BMSdb.dbc  MsgList=cell_temp_37_40  MsgName=cell_temp_37_40  MsgIDType=Standard (11-bit identifier)  MsgIdentifier=33  MsgLength=8  SignalInfo=cell37_temperature$8$16$2$2$1$0$1.000000e-03$-20$-20$80$#cell38_temperature$24$16$2$2$1$0$1.000000e-03$-20$-20$80$#cell39_temperature$40$16$2$2$1$0$1.000000e-03$-20$-20$80$#cell40_temperature$56$16$2$2$1$0$1.000000e-03$-20$-20$80$#  NSignals=4  StartBits=str2num('[int32(8);int32(24);int32(40);int32(56)]')  SignalSizes=str2num('[int32(16);int32(16);int32(16);int32(16)]')  ByteOrders=str2num('[int32(2);int32(2);int32(2);int32(2)]')  DataTypes=str2num('[int32(2);int32(2);int32(2);int32(2)]')  MultiplexTypes=str2num('[int32(1);int32(1);int32(1);int32(1)]')  MultiplexValues=str2num('[double(0);double(0);double(0);double(0)]')  Factors=str2num('[double(1.000000e-03);double(1.000000e-03);double(1.000000e-03);double(1.000000e-03)]')  Offsets=str2num('[double(-20);double(-20);double(-20);double(-20)]')  Minimums=str2num('[double(-20);double(-20);double(-20);double(-20)]')  Maximums=str2num('[double(80);double(80);double(80);double(80)]')  Remote=off
      settings: DataFormat=CANdb specified signals
  CAN Transmit : canlib/CAN Transmit  BlockHandle=597.0005  DeviceMenu=Kvaser Leaf Light v2 1 (Channel 1)  Device=Kvaser Leaf Light v2 1 (Channel 1)  ObjConstructor=canChannel('Kvaser', 'Leaf Light v2 1', 1)  EnablePeriodicTransmit=off  MessagePeriod=1.000
  CAN Transmit1 : canlib/CAN Transmit  BlockHandle=598.0005  DeviceMenu=Kvaser Leaf Light v2 1 (Channel 1)  Device=Kvaser Leaf Light v2 1 (Channel 1)  ObjConstructor=canChannel('Kvaser', 'Leaf Light v2 1', 1)  EnablePeriodicTransmit=off  MessagePeriod=1.000
  CAN Transmit2 : canlib/CAN Transmit  BlockHandle=599.0005  DeviceMenu=Kvaser Leaf Light v2 1 (Channel 1)  Device=Kvaser Leaf Light v2 1 (Channel 1)  ObjConstructor=canChannel('Kvaser', 'Leaf Light v2 1', 1)  EnablePeriodicTransmit=off  MessagePeriod=1.000
  CAN Transmit3 : canlib/CAN Transmit  BlockHandle=600.0005  DeviceMenu=Kvaser Leaf Light v2 1 (Channel 1)  Device=Kvaser Leaf Light v2 1 (Channel 1)  ObjConstructor=canChannel('Kvaser', 'Leaf Light v2 1', 1)  EnablePeriodicTransmit=off  MessagePeriod=1.000
  CAN Transmit4 : canlib/CAN Transmit  BlockHandle=601.0005  DeviceMenu=Kvaser Leaf Light v2 1 (Channel 1)  Device=Kvaser Leaf Light v2 1 (Channel 1)  ObjConstructor=canChannel('Kvaser', 'Leaf Light v2 1', 1)  EnablePeriodicTransmit=off  MessagePeriod=1.000
  CAN Transmit5 : canlib/CAN Transmit  BlockHandle=602.0005  DeviceMenu=Kvaser Leaf Light v2 1 (Channel 1)  Device=Kvaser Leaf Light v2 1 (Channel 1)  ObjConstructor=canChannel('Kvaser', 'Leaf Light v2 1', 1)  EnablePeriodicTransmit=off  MessagePeriod=1.000
  CAN Transmit6 : canlib/CAN Transmit  BlockHandle=603.0005  DeviceMenu=Kvaser Leaf Light v2 1 (Channel 1)  Device=Kvaser Leaf Light v2 1 (Channel 1)  ObjConstructor=canChannel('Kvaser', 'Leaf Light v2 1', 1)  EnablePeriodicTransmit=off  MessagePeriod=1.000
  CAN Transmit7 : canlib/CAN Transmit  BlockHandle=604.0005  DeviceMenu=Kvaser Leaf Light v2 1 (Channel 1)  Device=Kvaser Leaf Light v2 1 (Channel 1)  ObjConstructor=canChannel('Kvaser', 'Leaf Light v2 1', 1)  EnablePeriodicTransmit=off  MessagePeriod=1.000
  CAN Transmit8 : canlib/CAN Transmit  BlockHandle=605.0005  DeviceMenu=Kvaser Leaf Light v2 1 (Channel 1)  Device=Kvaser Leaf Light v2 1 (Channel 1)  ObjConstructor=canChannel('Kvaser', 'Leaf Light v2 1', 1)  EnablePeriodicTransmit=off  MessagePeriod=1.000
  CAN Transmit9 : canlib/CAN Transmit  BlockHandle=606.0005  DeviceMenu=Kvaser Leaf Light v2 1 (Channel 1)  Device=Kvaser Leaf Light v2 1 (Channel 1)  ObjConstructor=canChannel('Kvaser', 'Leaf Light v2 1', 1)  EnablePeriodicTransmit=off  MessagePeriod=1.000
  Demux{,1..9} (10 alike) : Demux
  Demux10 : Demux  Outputs=10
  wires:
  Demux5/4 -> CAN Pack5/4
  Demux5/1 -> CAN Pack5/1
  Demux5/2 -> CAN Pack5/2
  Demux5/3 -> CAN Pack5/3
  CAN Pack5/1 -> CAN Transmit5/1
  CAN Pack9/1 -> CAN Transmit9/1
  Demux9/4 -> CAN Pack9/4
  Demux9/1 -> CAN Pack9/1
  Demux9/2 -> CAN Pack9/2
  Demux8/1 -> CAN Pack8/1
  CAN Pack8/1 -> CAN Transmit8/1
  Demux8/3 -> CAN Pack8/3
  Demux8/2 -> CAN Pack8/2
  Demux8/4 -> CAN Pack8/4
  CAN Pack2/1 -> CAN Transmit2/1
  Demux1/4 -> CAN Pack1/4
  CAN Pack1/1 -> CAN Transmit1/1
  Demux1/1 -> CAN Pack1/1
  Demux1/2 -> CAN Pack1/2
  Demux1/3 -> CAN Pack1/3
  Demux4/1 -> CAN Pack4/1
  CAN Pack4/1 -> CAN Transmit4/1
  Demux4/3 -> CAN Pack4/3
  Demux4/2 -> CAN Pack4/2
  Demux4/4 -> CAN Pack4/4
  CAN Pack/1 -> CAN Transmit/1
  Demux/2 -> CAN Pack/2
  Demux/3 -> CAN Pack/3
  Demux/4 -> CAN Pack/4
  Demux6/2 -> CAN Pack6/2
  Demux6/4 -> CAN Pack6/4
  Demux6/3 -> CAN Pack6/3
  CAN Pack6/1 -> CAN Transmit6/1
  Demux6/1 -> CAN Pack6/1
  Demux3/2 -> CAN Pack3/2
  Demux3/1 -> CAN Pack3/1
  CAN Pack3/1 -> CAN Transmit3/1
  Demux3/4 -> CAN Pack3/4
  Demux3/3 -> CAN Pack3/3
  Demux7/2 -> CAN Pack7/2
  Demux7/4 -> CAN Pack7/4
  Demux7/3 -> CAN Pack7/3
  Demux7/1 -> CAN Pack7/1
  CAN Pack7/1 -> CAN Transmit7/1
  Demux10/1 -> Demux/1
  Demux10/2 -> Demux1/1
  Demux10/3 -> Demux2/1
  Demux10/4 -> Demux3/1
  Demux10/5 -> Demux4/1
  Demux10/6 -> Demux5/1
  Demux10/7 -> Demux6/1
  Demux10/8 -> Demux7/1
  Demux10/9 -> Demux8/1
  Demux10/10 -> Demux9/1
  cell_temperatures/1 -> Demux10/1
  Demux/1 -> CAN Pack/1
  Demux9/3 -> CAN Pack9/3
  Demux2/1 -> CAN Pack2/4
  Demux2/2 -> CAN Pack2/1
  Demux2/3 -> CAN Pack2/2
  Demux2/4 -> CAN Pack2/3
